simulink model "cssim_pds_demo"  (Simulink 6.5)
settings: Solver=ode45  StartTime=0.0  StopTime=20  RelTol=1e-3
libraries: truetime x1
settings Model: Creator=David  LastModifiedBy=Administrator
settings DataIOCC: LimitDataPoints=off  SignalLoggingName=sigsOut
settings OptimizationCC: InlineInvariantSignals=on
settings DebuggingCC: SolverPrmCheckMsg=none  MultiTaskDSMMsg=warning  MultiTaskCondExecSysMsg=none  StrictBusMsg=None
settings HardwareCC: TargetUnknown=on
settings RTWCC: IncludeERTFirstTime=on

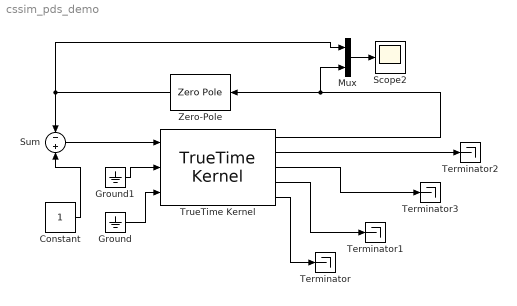
== system cssim_pds_demo ==
  Constant : Constant  Value=1  OutDataType=sfix(16)  ConRadixGroup=Use specified scaling  OutScaling=2^0  SampleTime=inf  FramePeriod=inf
  Ground : Ground
  Ground1 : Ground
  Mux : Mux  Inputs=2
  Scope2 : Scope
  Sum : Sum  Inputs=-|+
  Terminator{,1..3} (4 alike) : Terminator
  TrueTime Kernel : truetime/TrueTime Kernel  SystemSampleTime=-1  sfun=simple_init  args=0  battery=off  clockdrift=0  clockoffset=0
  Zero-Pole : ZeroPole  Orientation=left  Zeros=[]  Poles=[0 -1 -1]
  wires:
  TrueTime Kernel/5 -> Terminator/1
  Ground/1 -> TrueTime Kernel/3
  Ground1/1 -> TrueTime Kernel/2
  TrueTime Kernel/2 -> Terminator2/1
  Mux/1 -> Scope2/1
  TrueTime Kernel/4 -> Terminator1/1
  Zero-Pole/1 -> Mux/1, Sum/1
  TrueTime Kernel/1 -> Zero-Pole/1, Mux/2
  Sum/1 -> TrueTime Kernel/1
  Constant/1 -> Sum/2
  TrueTime Kernel/3 -> Terminator3/1
